simulink model "Closed_loop_Interferometer_v5_double_int"  (R2019b)
settings: Solver=ode3  StartTime=0.0  StopTime=0.5  FixedStep=0.00001  RelTol=1e-3  EnableMultiTasking=on
InitFcn:
  | clear all
  | close all
  | clc
  | 
  | %control interferometer
  | A1=0.3;
  | V1=0.666;
  | %sensor interferometer
  | A2=0.17;
  | V2=0.4705;
  | timer=0.1;
  | 
  | op_sensor = 0;
  | op_control = op_sensor + 0*pi;
  | control_set_point = 0*A1*V1;
StopFcn:
  | set(groot,'defaultAxesTickLabelInterpreter','latex')
  | set(groot,'defaultLegendInterpreter','latex')
  | xc = 0.3;
  | 
  | %%%%
  | figure('Units','centimeter','Position',[0 0 20 30])
  | 
  | 
  | subplot(6,1,1)
  | plot(cleanSignal,'Color',[xc,xc,xc])
  | xlim([0 inf])
  | %ylim([-1 1])
  | xlabel('Time [s]','Interpreter','latex', 'FontSize', 10)
  | ylabel({'Input signal' ;'[rad]'},'Interpreter','latex', 'FontSize', 10)
  | title('')
  | grid
  | 
  | subplot(6,1,2)
  | plot(input,'Color',[xc,xc,xc])
  | %ylim([0.8*min(input.data) 1.2*max(input.data)])
  | xlim([0 inf])
  | xlabel('Time [s]','Interpreter','latex', 'FontSize', 10)
  | ylabel({'Input signal w/';'disturbances [rad]'},'Interpreter','latex', 'FontSize', 10)
  | title('')
  | grid
  | 
  | 
  | subplot(6,1,3)
  | plot(signFunc,'Color',[xc,xc,xc],'LineWidth',0.1)
  | ylim([-1.2 1.2])
  | xlim([0 inf])
  | xlabel('Time [s]','Interpreter','latex', 'FontSize', 10)
  | ylabel({'Sign function';'output [V]'},'Interpreter','latex', 'FontSize', 10)
  | title('')
  | grid
  | 
  | 
  | subplot(6,1,4)
  | plot(controlSignal,'Color',[xc,xc,xc])
  | %ylim([-5 0.2])
  | xlim([0 inf])
  | xlabel('Time [s]','Interpreter','latex', 'FontSize', 10)
  | ylabel({'Feedback control';'signal [rad]' },'Interpreter','latex', 'FontSize', 10)
  | title('')
  | grid minor
  | 
  | subplot(6,1,5)
  | plot(output,'Color',[xc,xc,xc])
  | xline(timer,'Color',[41/256 128/256 185/256],'LineWidth',1.5)
  | ylim([-1.2*(A1+(A1*V1)) 1.2*(A1+(A1*V1)) ])
  | xlim([0 inf])
  | xlabel('Time [s]','Interpreter','latex', 'FontSize', 10)
  | ylabel({'Control';'Interferometer';'[rad]'},'Interpreter','latex', 'FontSize', 10) %rad or V, A=1W/V
  | title('')
  | legend(['Start operation point = ',num2str(op_control),'[rad]', '   Setpoint = ',num2str(control_set_point )],'Control start','Location','Best')
  | grid
  | 
  | subplot(6,1,6)
  | plot(output2,'Color',[xc,xc,xc])
  | xline(timer,'Color',[41/256 128/256 185/256],'LineWidth',1.5)
  | ylim([-1.2*(A2+(A2*V2)) 1.2*(A2+(A2*V2)) ])
  | xlim([0 inf])
  | xlabel('Time [s]','Interpreter','latex', 'FontSize', 10)
  | ylabel({'Sensor';'Interferometer';' [rad]'},'Interpreter','latex', 'FontSize', 10) %rad or V, A=1W/V
  | title('')
  | legend(['Operation point = ',num2str(op_sensor),'[rad]'],'Control start','Location','Best')
  | grid
  | 
  | %figure
  | %plot(lowpass,'Color',[xc,xc,xc])
  | 
  | cd 'D:\Users\Stinky\Google Drive\ITA\Codes\MATLAB'
  | 
  | print('test','-dpdf'); %-dpng , -depsc, -tiff, -dpdf
undefined symbols (not defined in the file or in its folder): sgn
libraries: simulink x1, dsparch4 x1
settings Model: Creator=Roberta Martin  LastModifiedBy=Stinky
settings DataIOCC: LimitDataPoints=on  SaveFormat=Array  ReturnWorkspaceOutputs=off
settings OptimizationCC: LifeSpan=inf
settings DebuggingCC: UnderspecifiedInitializationDetection=Classic  MergeDetectMultiDrivingBlocksExec=none  SolverPrmCheckMsg=warning  AllowSymbolicDim=off  SFUnexpectedBacktrackingDiag=warning  SFNoUnconditionalDefaultTransitionDiag=warning  SFExecutionAtInitializationDiag=none  ArithmeticOperatorsInVariantConditions=warning
settings HardwareCC: ProdBitPerPointer=32  ProdBitPerSizeT=32  ProdBitPerPtrDiffT=32  ProdLargestAtomicFloat=None  ProdIntDivRoundTo=Undefined  ProdEndianess=Unspecified  ProdWordSize=32  ProdHWDeviceType=32-bit Generic
settings ModelReferenceCC: PropagateSignalLabelsOutOfModel=off
settings SFSimCC: SimUseLocalCustomCode=off  CustomCodeUndefinedFunction=UseInterfaceOnly
settings RTWCC: RTWUseLocalCustomCode=off
settings CodeAppCC: StateflowObjectComments=on
settings GRTTargetCC: TargetLangStandard=C89/C90 (ANSI)  GeneratePreprocessorConditionals=Disable all
settings ConfigComp: CovMetricSettings=dw  CovHtmlReporting=on  CovSaveCumulativeToWorkspaceVar=on  CovSaveSingleToWorkspaceVar=on  CovExternalEMLEnable=off
settings SimscapeCC: SimscapeNormalizeSystem=off

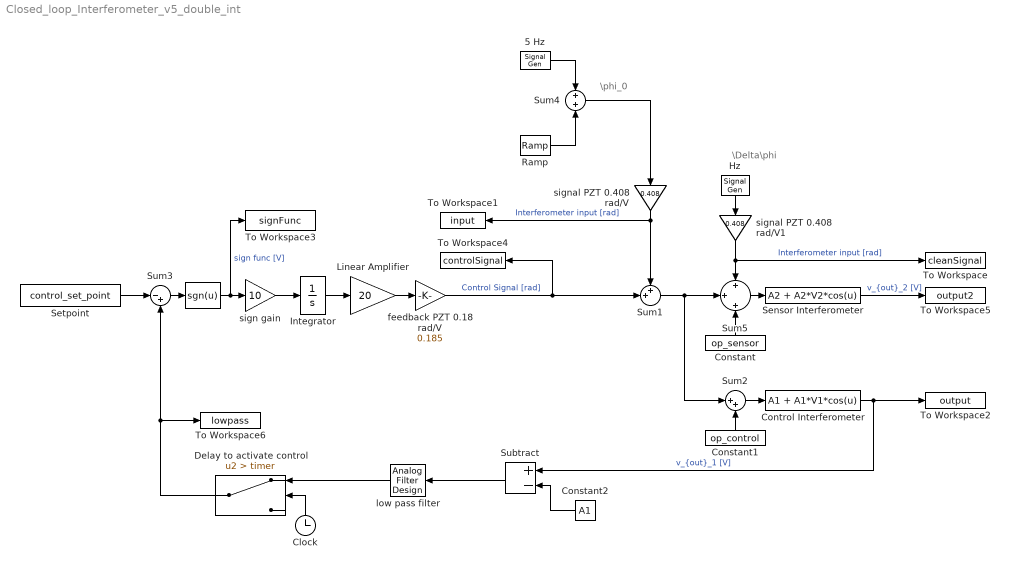
== system Closed_loop_Interferometer_v5_double_int ==
  note: \phi_0
  note: \Delta\phi
  " " : Fcn  Expr=sgn(u)
  " 5 Hz" : SignalGenerator  Amplitude=2  Frequency=5
  Clock : Clock
  Constant : Constant  Value=op_sensor
  Constant1 : Constant  Value=op_control
  Constant2 : Constant  Value=A1
  Control Interferometer : Fcn  Expr=A1 + A1*V1*cos(u)
  Delay to activate control : Switch  Criteria=u2 > Threshold  Threshold=timer
  "Hz " : SignalGenerator  Amplitude=2  Frequency=30
  Integrator : Integrator  LimitOutput=on  UpperSaturationLimit=15  LowerSaturationLimit=-15
  Linear Amplifier : Gain  Gain=20
  Ramp : simulink/Sources/Ramp  slope=10  start=0  InitialOutput=0
  Sensor Interferometer : Fcn  Expr=A2 + A2*V2*cos(u)
  Setpoint : Constant  Value=control_set_point
  Subtract : Sum  Inputs=+-
  Sum1 : Sum  Inputs=++|
  Sum2 : Sum  Inputs=|++
  Sum3 : Sum  Inputs=|-+
  Sum4 : Sum  Inputs=+|+
  Sum5 : Sum  Inputs=+|+|+
  To Workspace : ToWorkspace  VariableName=cleanSignal  SaveFormat=Timeseries  SampleTime=-1
  To Workspace1 : ToWorkspace  VariableName=input  SaveFormat=Timeseries  SampleTime=-1
  To Workspace2 : ToWorkspace  VariableName=output  SaveFormat=Timeseries  SampleTime=-1
  To Workspace3 : ToWorkspace  VariableName=signFunc  SaveFormat=Timeseries  SampleTime=-1
  To Workspace4 : ToWorkspace  VariableName=controlSignal  SaveFormat=Timeseries  SampleTime=-1
  To Workspace5 : ToWorkspace  VariableName=output2  SaveFormat=Timeseries  SampleTime=-1
  To Workspace6 : ToWorkspace  VariableName=lowpass  SaveFormat=Timeseries  SampleTime=-1
  feedback PZT 0.18 rad/V : Gain  Gain=0.185
  low pass filter : dsparch4/Analog Filter Design  method=Butterworth  filttype=Lowpass  N=1  Wlo=1000*2*pi  Whi=80  Rp=2  Rs=40
  sign gain : Gain  Gain=10
  signal PZT 0.408 rad/V : Gain  Gain=0.408
  signal PZT 0.408 rad/V1 : Gain  Gain=0.408
  wires:
  Control Interferometer/1 -> Subtract/1, To Workspace2/1  "v_{out}_1 [V]"
  Sum1/1 -> Sum2/1, Sum5/2
  Linear Amplifier/1 -> feedback PZT 0.18 rad/V/1
  signal PZT 0.408 rad/V/1 -> Sum1/1, To Workspace1/1  "Interferometer input [rad]"
  Sum3/1 -> " "/1
  Setpoint/1 -> Sum3/1
  sign gain/1 -> Integrator/1
  Clock/1 -> Delay to activate control/2
  low pass filter/1 -> Delay to activate control/1
  " 5 Hz"/1 -> Sum4/1
  Ramp/1 -> Sum4/2
  " "/1 -> To Workspace3/1, sign gain/1  "sign func [V]"
  Integrator/1 -> Linear Amplifier/1
  Sum5/1 -> Sensor Interferometer/1
  Sensor Interferometer/1 -> To Workspace5/1  "v_{out}_2 [V]"
  Delay to activate control/1 -> To Workspace6/1, Sum3/2
  Sum4/1 -> signal PZT 0.408 rad/V/1
  "Hz "/1 -> signal PZT 0.408 rad/V1/1
  Constant/1 -> Sum5/3
  signal PZT 0.408 rad/V1/1 -> To Workspace/1, Sum5/1  "Interferometer input [rad]"
  Sum2/1 -> Control Interferometer/1
  Constant1/1 -> Sum2/2
  feedback PZT 0.18 rad/V/1 -> To Workspace4/1, Sum1/2  "Control Signal [rad]"
  Subtract/1 -> low pass filter/1
  Constant2/1 -> Subtract/2
